simulink model "R3GDL"  (Simulink 9.0)
settings: Solver=ode45  StartTime=0.0  StopTime=Tsim  MaxStep=1e-3  RelTol=1e-3  EnableMultiTasking=on
values from neighbouring files (symbols this model uses):
  duracion = 1    [Controladores.m]    (also in GTCL_R3GDL.m = in(9))
  Kd = Kp*tau    [Control_Disc.m]    (also in Control_PID.m; Controladores.m; PD_Feedforward.m; dsgn_PD.m = Kp.*Td)
  Ki = [0 0 0]    [Control_Disc.m]    (also in Control_PID.m = [0 0 0]'; Controladores.m; PD_Feedforward.m; dsgn_PD.m = Kp./Ti)
  Kp = [7.4989e+04 1.4125e+05 1.5488e+04]    [Control_Disc.m]    (also in Control_PID.m = [7.4989e+04 1.4125e+05 1.5488e+04]'; Controladores.m; PD_Feedforward.m; dsgn_PD.m = [2.1312e+06 8.4844e+05 4.5042e+05])
  n = 5    [Controladores.m]    (also in GTCL_R3GDL.m = in(7))
  R1 = 1    [ModeloDinamico_R3GDL.m]    (also in PD_Feedforward.m)
  R2 = 1    [ModeloDinamico_R3GDL.m]    (also in PD_Feedforward.m)
  R3 = 1    [ModeloDinamico_R3GDL.m]    (also in PD_Feedforward.m)
  t_ini = 0.5    [Controladores.m]
  XYZfin = CinematicaDirecta([pi 3*pi/4 -pi/5])    [Controladores.m]    (also in GTCL_R3GDL.m = [in(4) in(5) in(6)]')
  XYZini = CinematicaDirecta([0 0 0])    [Controladores.m]
undefined symbols (not defined in the file or in its folder): Ts
settings Model: Creator=mortega  LastModifiedBy=Raúl  ExtModeTrigMode=oneshot  ExtModeArmWhenConnect=off
settings DataIOCC: SignalLoggingSaveFormat=ModelDataLogs
settings OptimizationCC: BlockReduction=off  BooleanDataType=off  ExpressionDepthLimit=2147483647  InitFltsAndDblsToZero=on
settings DebuggingCC: SaveWithParameterizedLinksMsg=none  SignalResolutionControl=TryResolveAllWithWarning  MultiTaskDSMMsg=warning  MultiTaskCondExecSysMsg=none  FcnCallInpInsideContextMsg=warning  StateNameClashWarn=warning  StrictBusMsg=None
settings HardwareCC: TargetUnknown=on
settings GRTTargetCC: TargetFcnLib=ansi_tfl_tmw.mat  CombineOutputUpdateFcns=off  GRTInterface=on

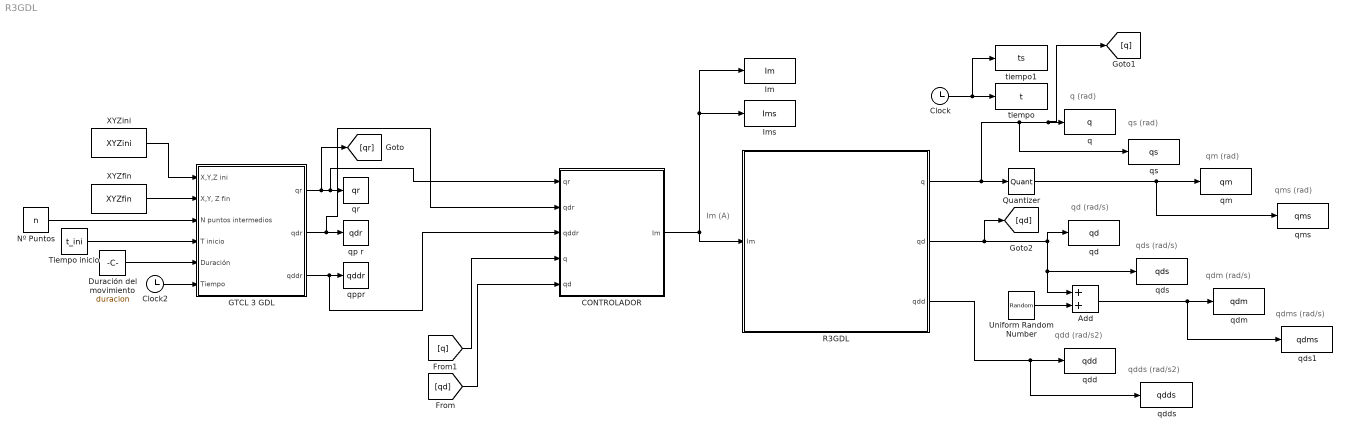
== system R3GDL ==
  note: Im (A)
  note: q (rad)
  note: qd (rad/s)
  note: qdd (rad/s2)
  note: qs (rad)
  note: qds (rad/s)
  note: qdds (rad/s2)
  note: qm (rad)
  note: qms (rad)
  note: qdm (rad/s)
  note: qdms (rad/s)
  Add : Sum
  "CONTROLADOR " : Subsystem
  Clock : Clock
  Clock2 : Clock
  Duración del movimiento : Constant  Value=duracion
  GTCL 3 GDL : Subsystem
  Im : ToWorkspace  VariableName=Im  SampleTime=-1
  Ims : ToWorkspace  VariableName=Ims  SampleTime=Ts
  Nº Puntos : Constant  Value=n
  Quantizer : Quantizer  QuantizationInterval=2*pi/512./[R1 R2 R3]
  R3GDL : Subsystem  mask(Control y Programación de Robots (4 GIERM)){NGrupo=3, q1_ini=0, q2_ini=0, q3_ini=0, Bl_q1=off, Bl_q2=off, Bl_q3=off, AccionamientoDirecto=on}
      mask prompts: NGrupo "Nº de GRUPO"; q1_ini "q1 inicial  (rad)"; q2_ini "q2 inicial (rad)"; q3_ini "q3_inicial (rad)"; Bl_q1 "Bloqueo q1"; Bl_q2 "Bloqueo q2"; Bl_q3 "Bloqueo q3"; AccionamientoDirecto "Accionamiento directo"
      mask help: Robot de 3 grados de libertad RRR
      mask Display:
      | image(imread('R3GDL_RRR.JPG'));
      | port_label('output', 1, 'q');
      | port_label('output', 2, 'qd');
      | port_label('output', 3, 'qdd');
      | port_label('input', 1, 'Im')
  Tiempo inicio : Constant  Value=t_ini
  Uniform Random Number : UniformRandomNumber  Minimum=-1500*2*pi/60./[R1 R2 R3]*0.02  Maximum=1500*2*pi/60./[R1 R2 R3]*0.02  SampleTime=Ts/10
  XYZfin : Constant  Value=XYZfin
  XYZini : Constant  Value=XYZini
  q : ToWorkspace  VariableName=q  SampleTime=-1
  qd : ToWorkspace  VariableName=qd  SampleTime=-1
  qdd : ToWorkspace  VariableName=qdd  SampleTime=-1
  qdds : ToWorkspace  VariableName=qdds  SampleTime=Ts
  qdm : ToWorkspace  VariableName=qdm  SampleTime=-1
  qds : ToWorkspace  VariableName=qds  SampleTime=Ts
  qds1 : ToWorkspace  VariableName=qdms  SampleTime=Ts
  qm : ToWorkspace  VariableName=qm  SampleTime=-1
  qms : ToWorkspace  VariableName=qms  SampleTime=Ts
  qp r : ToWorkspace  VariableName=qdr  SampleTime=-1
  qppr : ToWorkspace  VariableName=qddr  SampleTime=-1
  qr : ToWorkspace  VariableName=qr  SampleTime=-1
  qs : ToWorkspace  VariableName=qs  SampleTime=Ts
  tiempo : ToWorkspace  VariableName=t  SampleTime=-1
  tiempo1 : ToWorkspace  VariableName=ts  SampleTime=Ts
  wires:
  Clock/1 -> tiempo1/1, tiempo/1
  Add/1 -> qdm/1, qds1/1
  Uniform Random Number/1 -> Add/2
  Quantizer/1 -> qm/1, qms/1
  R3GDL/3(qdd) -> qdd/1, qdds/1
  R3GDL/2(qd) -> [qd], qds/1, Add/1, qd/1
  R3GDL/1(q) -> Quantizer/1, [q], q/1, qs/1
  "CONTROLADOR "/1("Im  ") -> R3GDL/1(Im), Ims/1, Im/1
  Nº Puntos/1 -> GTCL 3 GDL/3(N puntos intermedios)
  GTCL 3 GDL/2(qdr) -> qp r/1, "CONTROLADOR "/2(qdr)
  Duración del movimiento/1 -> GTCL 3 GDL/5(Duración)
  Clock2/1 -> GTCL 3 GDL/6(Tiempo)
  GTCL 3 GDL/1(qr) -> [qr], qr/1, "CONTROLADOR "/1(qr)
  GTCL 3 GDL/3(qddr) -> qppr/1, "CONTROLADOR "/3(qddr)
  Tiempo inicio/1 -> GTCL 3 GDL/4(T inicio)
  XYZini/1 -> GTCL 3 GDL/1(X,Y,Z ini)
  XYZfin/1 -> GTCL 3 GDL/2("X,Y, Z fin")
  [q] -> "CONTROLADOR "/4(q)
  [qd] -> "CONTROLADOR "/5(qd)

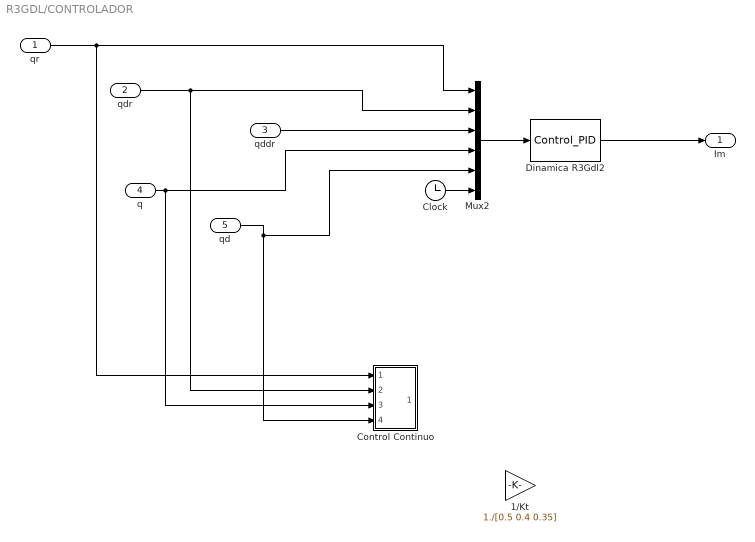
== system R3GDL/CONTROLADOR  ==
  qr : Inport
  qdr : Inport  Port=2
  qddr : Inport  Port=3
  q : Inport  Port=4
  qd : Inport  Port=5
  "1/Kt " : Gain  Gain=1./[0.5 0.4 0.35]
  Clock : Clock
  "Control Continuo " : Subsystem
  Dinamica R3Gdl2 : MATLABFcn  MATLABFcn=Control_PID  SampleTime=1e-3
  Mux2 : Mux  Inputs=6
  "Im  " : Outport
  wires:
  Clock/1 -> Mux2/6
  qd/1 -> Mux2/5, "Control Continuo "/4(In4)
  q/1 -> Mux2/4, "Control Continuo "/3(In3)
  qddr/1 -> Mux2/3
  qdr/1 -> Mux2/2, "Control Continuo "/2(In2)
  qr/1 -> Mux2/1, "Control Continuo "/1(In1)
  Mux2/1 -> Dinamica R3Gdl2/1
  Dinamica R3Gdl2/1 -> "Im  "/1

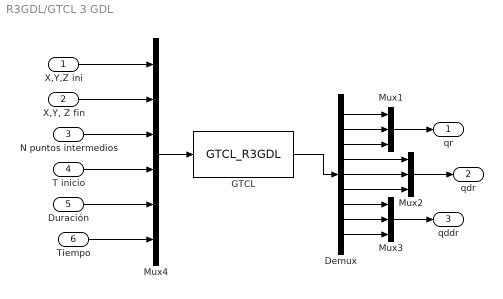
== system R3GDL/GTCL 3 GDL ==
  X,Y,Z ini : Inport
  "X,Y, Z fin" : Inport  Port=2
  N puntos intermedios : Inport  Port=3
  T inicio : Inport  Port=4
  Duración : Inport  Port=5
  Tiempo : Inport  Port=6
  Demux : Demux  Outputs=9
  GTCL : MATLABFcn  MATLABFcn=GTCL_R3GDL  OutputDimensions=9
  Mux1 : Mux  Inputs=3
  Mux2 : Mux  Inputs=3
  Mux3 : Mux  Inputs=3
  Mux4 : Mux  Inputs=6
  qr : Outport
  qdr : Outport  Port=2
  qddr : Outport  Port=3
  wires:
  Demux/9 -> Mux3/3
  Demux/8 -> Mux3/2
  Demux/7 -> Mux3/1
  Mux3/1 -> qddr/1
  Demux/6 -> Mux2/3
  Demux/5 -> Mux2/2
  Demux/4 -> Mux2/1
  Mux2/1 -> qdr/1
  Demux/3 -> Mux1/3
  Demux/2 -> Mux1/2
  Demux/1 -> Mux1/1
  GTCL/1 -> Demux/1
  Tiempo/1 -> Mux4/6
  Duración/1 -> Mux4/5
  T inicio/1 -> Mux4/4
  N puntos intermedios/1 -> Mux4/3
  "X,Y, Z fin"/1 -> Mux4/2
  X,Y,Z ini/1 -> Mux4/1
  Mux4/1 -> GTCL/1
  Mux1/1 -> qr/1

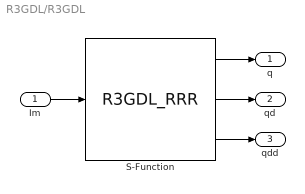
== system R3GDL/R3GDL ==
  Im : Inport
  S-Function : S-Function  FunctionName=R3GDL_RRR  Parameters=[q1_ini; q2_ini; q3_ini]; [Bl_q1; Bl_q2; Bl_q3]; AccionamientoDirecto; NGrupo  SFunctionDeploymentMode=off  EnableBusSupport=off
  q : Outport
  qd : Outport  Port=2
  qdd : Outport  Port=3
  wires:
  Im/1 -> S-Function/1
  S-Function/1 -> q/1
  S-Function/2 -> qd/1
  S-Function/3 -> qdd/1

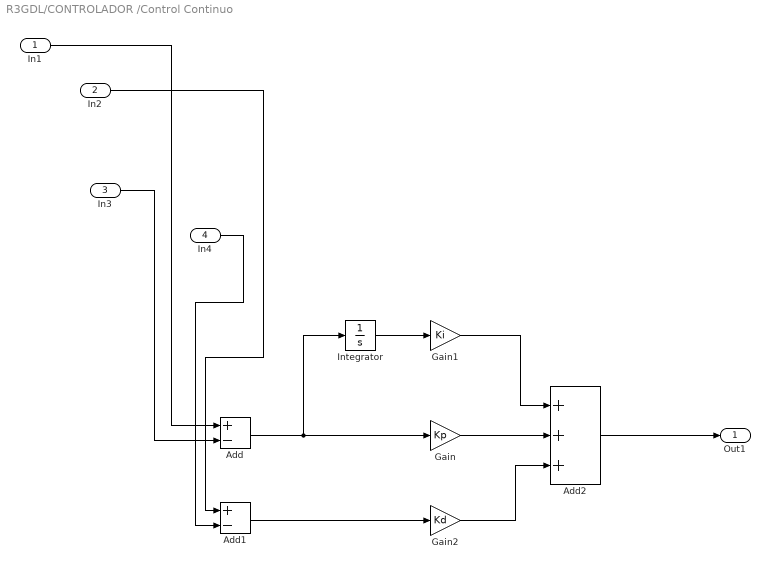
== system R3GDL/CONTROLADOR /Control Continuo  ==
  In1 : Inport
  In2 : Inport  Port=2
  In3 : Inport  Port=3
  In4 : Inport  Port=4
  Add : Sum  Inputs=+-
  Add1 : Sum  Inputs=+-
  Add2 : Sum  Inputs=+++
  Gain : Gain  Gain=Kp
  Gain1 : Gain  Gain=Ki
  Gain2 : Gain  Gain=Kd
  Integrator : Integrator
  Out1 : Outport
  wires:
  In3/1 -> Add/2
  Add2/1 -> Out1/1
  In1/1 -> Add/1
  In4/1 -> Add1/2
  In2/1 -> Add1/1
  Gain1/1 -> Add2/1
  Gain/1 -> Add2/2
  Add1/1 -> Gain2/1
  Gain2/1 -> Add2/3
  Integrator/1 -> Gain1/1
  Add/1 -> Integrator/1, Gain/1
